simulink model "hh_ap"  (R2020b)
settings: Solver=VariableStepAuto  StartTime=0.0  StopTime=10.0  RelTol=1e-3
values from neighbouring files (symbols this model uses):
  capa = 1    [hh_ap_source.m]
  E_K = -12    [hh_ap_source.m]
  E_L = 10.613    [hh_ap_source.m]
  E_Na = 115    [hh_ap_source.m]
  G_K_max = 36    [hh_ap_source.m]
  G_L = 0.3    [hh_ap_source.m]
  G_Na_max = 120    [hh_ap_source.m]
  h0 = 1    [hh_ap_source.m]
  m0 = 0    [hh_ap_source.m]
  n0 = 0    [hh_ap_source.m]
  V0 = 0    [hh_ap_source.m]
settings Model: Creator=haedo  LastModifiedBy=haedo

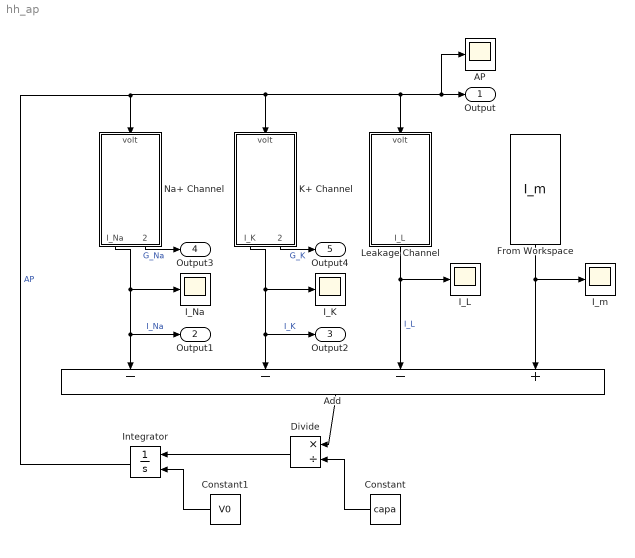
== system hh_ap ==
  AP : Scope
  Add : Sum  Inputs=---+
  Constant : Constant  Value=capa
  Constant1 : Constant  Value=V0
  Divide : Product  Inputs=*/
  From Workspace : FromWorkspace  VariableName=I_m
  I_K : Scope
  I_L : Scope
  I_Na : Scope
  I_m : Scope
  Integrator : Integrator  InitialConditionSource=external
  K+ Channel : Subsystem
  Leakage Channel : Subsystem
  Na+ Channel : Subsystem
  Output : Outport  VectorParamsAs1DForOutWhenUnconnected=off
  Output1 : Outport  Port=2  VectorParamsAs1DForOutWhenUnconnected=off
  Output2 : Outport  Port=3  VectorParamsAs1DForOutWhenUnconnected=off
  Output3 : Outport  Port=4  VectorParamsAs1DForOutWhenUnconnected=off
  Output4 : Outport  Port=5  VectorParamsAs1DForOutWhenUnconnected=off
  wires:
  Leakage Channel/1(I_L) -> I_L/1, Add/3  "I_L"
  Na+ Channel/2(G_Na_out) -> Output3/1  "G_Na"
  K+ Channel/2(G_K_out) -> Output4/1  "G_K"
  Constant1/1 -> Integrator/2
  Divide/1 -> Integrator/1
  Add/1 -> Divide/1
  Constant/1 -> Divide/2
  Na+ Channel/1(I_Na) -> I_Na/1, Output1/1, Add/1  "I_Na"
  Integrator/1 -> Na+ Channel/1(volt), AP/1, Output/1, Leakage Channel/1(volt), K+ Channel/1(volt)  "AP"
  K+ Channel/1(I_K) -> I_K/1, Output2/1, Add/2  "I_K"
  From Workspace/1 -> Add/4, I_m/1

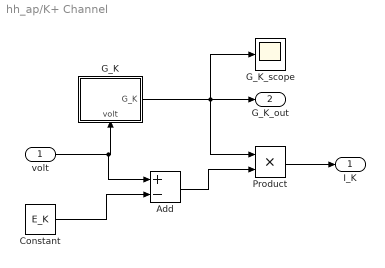
== system hh_ap/K+ Channel ==
  volt : Inport
  Add : Sum  Inputs=+-
  Constant : Constant  Value=E_K
  G_K : Subsystem
      settings: PortSchema="{\"entries\":[{\"content\":{\"sides\":[{\"content\":{\"connectorIds\":[]},\"type\":\"ConnectorPlacement.EquallySpacedRectSide\",\"uuid\":\"c632c91d-1676-4ce6-ab06-0028f8692ea5\"},{\"content\":{\"connectorIds\":[\"Out1\"],\"side\":\"RIGHT\"},\"type\":\"ConnectorPlacement.EquallySpacedRectSide\",\"uuid\":\"77b5085d-448e-4fc4-839b-3922e0b13526\"},{\"content\":{\"connectorIds\":[],\"side\":\"TOP\"},\"type\":\"ConnectorPlacement.EquallySpacedRectSide\",\"uuid\":\"dde0a616-523c-44d7-906e-d12cd1b401cf\"},{\"content\":{\"connectorIds\":[\"In1\"],\"side\":\"BOTTOM\"},\"type\":\"ConnectorPlacement.EquallySpacedRectSide\",\"uuid\":\"6c2ebf81-88aa-4156-83e6-a680f4cc31d9\"},{\"content\":{\"connectorIds\":[],\"side\":\"HIDDEN\"},\"type\":\"ConnectorPlacement.EquallySpacedRectSide\",\"uuid\":\"db869b89-d2b9-4524-8487-965b7fee0f2a\"}]},\"type\":\"ConnectorPlacement.EquallySpacedConnector\",\"uuid\":\"378f1207-81e2-4c7e-8dbf-20f9b4c806d5\"}],\"packageUris\":[\"http://schema.mathworks.com/mf0/Connector/R2020b\"],\"version\":\"1.0\"}"
  G_K_scope : Scope
  Product : Product
  I_K : Outport  VectorParamsAs1DForOutWhenUnconnected=off
  G_K_out : Outport  Port=2  VectorParamsAs1DForOutWhenUnconnected=off
  wires:
  volt/1 -> Add/1, G_K/1(volt)
  Constant/1 -> Add/2
  G_K/1(G_K) -> G_K_scope/1, G_K_out/1, Product/1
  Add/1 -> Product/2
  Product/1 -> I_K/1

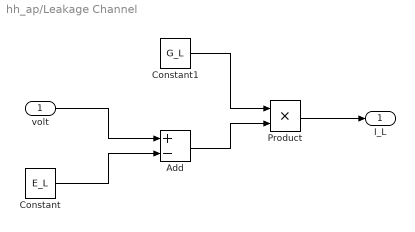
== system hh_ap/Leakage Channel ==
  volt : Inport
  Add : Sum  Inputs=+-
  Constant : Constant  Value=E_L
  Constant1 : Constant  Value=G_L
  Product : Product
  I_L : Outport  VectorParamsAs1DForOutWhenUnconnected=off
  wires:
  volt/1 -> Add/1
  Constant/1 -> Add/2
  Add/1 -> Product/2
  Constant1/1 -> Product/1
  Product/1 -> I_L/1

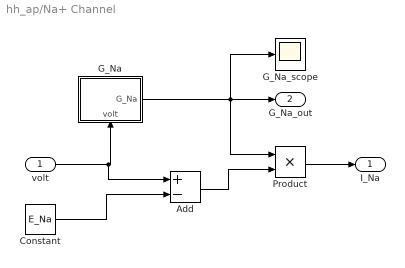
== system hh_ap/Na+ Channel ==
  volt : Inport
  Add : Sum  Inputs=+-
  Constant : Constant  Value=E_Na
  G_Na : Subsystem
      settings: PortSchema="{\"entries\":[{\"content\":{\"sides\":[{\"content\":{\"connectorIds\":[]},\"type\":\"ConnectorPlacement.EquallySpacedRectSide\",\"uuid\":\"c632c91d-1676-4ce6-ab06-0028f8692ea5\"},{\"content\":{\"connectorIds\":[\"Out1\"],\"side\":\"RIGHT\"},\"type\":\"ConnectorPlacement.EquallySpacedRectSide\",\"uuid\":\"77b5085d-448e-4fc4-839b-3922e0b13526\"},{\"content\":{\"connectorIds\":[],\"side\":\"TOP\"},\"type\":\"ConnectorPlacement.EquallySpacedRectSide\",\"uuid\":\"dde0a616-523c-44d7-906e-d12cd1b401cf\"},{\"content\":{\"connectorIds\":[\"In1\"],\"side\":\"BOTTOM\"},\"type\":\"ConnectorPlacement.EquallySpacedRectSide\",\"uuid\":\"c48f64ba-ba8f-42a4-9bef-aedab16ae96a\"},{\"content\":{\"connectorIds\":[],\"side\":\"HIDDEN\"},\"type\":\"ConnectorPlacement.EquallySpacedRectSide\",\"uuid\":\"db869b89-d2b9-4524-8487-965b7fee0f2a\"}]},\"type\":\"ConnectorPlacement.EquallySpacedConnector\",\"uuid\":\"378f1207-81e2-4c7e-8dbf-20f9b4c806d5\"}],\"packageUris\":[\"http://schema.mathworks.com/mf0/Connector/R2020b\"],\"version\":\"1.0\"}"
  G_Na_scope : Scope
  Product : Product
  I_Na : Outport  VectorParamsAs1DForOutWhenUnconnected=off
  G_Na_out : Outport  Port=2  VectorParamsAs1DForOutWhenUnconnected=off
  wires:
  volt/1 -> Add/1, G_Na/1(volt)
  Constant/1 -> Add/2
  G_Na/1(G_Na) -> G_Na_scope/1, G_Na_out/1, Product/1
  Add/1 -> Product/2
  Product/1 -> I_Na/1

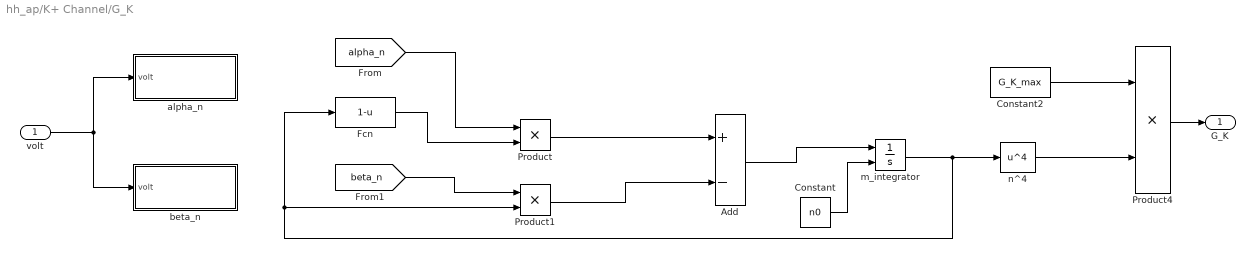
== system hh_ap/K+ Channel/G_K ==
  volt : Inport
  Add : Sum  Inputs=+-
  Constant : Constant  Value=n0
  Constant2 : Constant  Value=G_K_max
  Fcn : Fcn  Expr=1-u
  Product : Product
  Product1 : Product
  Product4 : Product
  alpha_n : Subsystem
  beta_n : Subsystem
  m_integrator : Integrator  InitialConditionSource=external
  n^4 : Fcn  Expr=u^4
  G_K : Outport
  wires:
  volt/1 -> alpha_n/1(volt), beta_n/1(volt)
  Product/1 -> Add/1
  [beta_n] -> Product1/1
  Add/1 -> m_integrator/1
  Product1/1 -> Add/2
  [alpha_n] -> Product/1
  Constant2/1 -> Product4/1
  n^4/1 -> Product4/2
  Product4/1 -> G_K/1
  m_integrator/1 -> n^4/1, Fcn/1, Product1/2
  Constant/1 -> m_integrator/2
  Fcn/1 -> Product/2

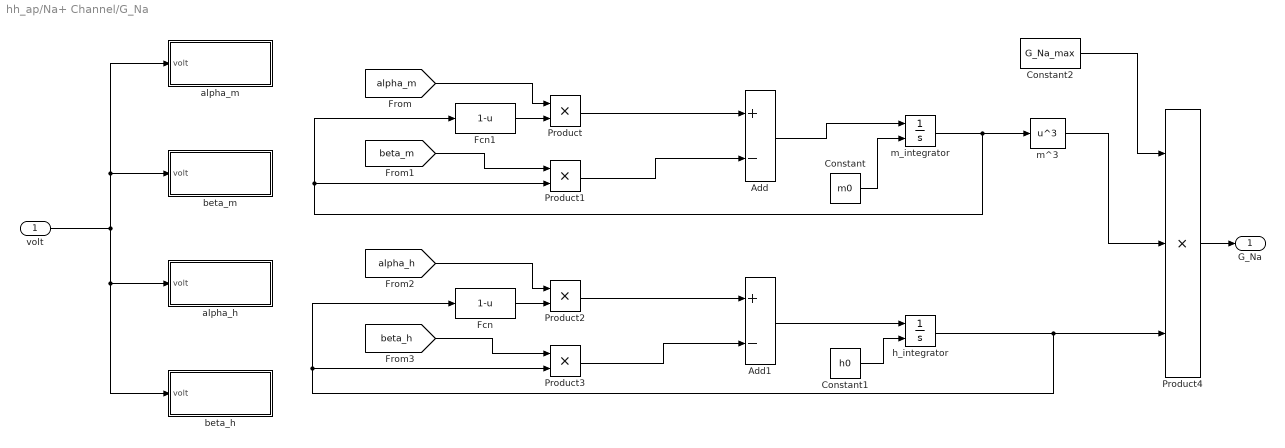
== system hh_ap/Na+ Channel/G_Na ==
  volt : Inport
  Add : Sum  Inputs=+-
  Add1 : Sum  Inputs=+-
  Constant : Constant  Value=m0
  Constant1 : Constant  Value=h0
  Constant2 : Constant  Value=G_Na_max
  Fcn : Fcn  Expr=1-u
  Fcn1 : Fcn  Expr=1-u
  Product{,1..3} (4 alike) : Product
  Product4 : Product  Inputs=3
  alpha_h : Subsystem
  alpha_m : Subsystem
  beta_h : Subsystem
  beta_m : Subsystem
  h_integrator : Integrator  InitialConditionSource=external
  m^3 : Fcn  Expr=u^3
  m_integrator : Integrator  InitialConditionSource=external
  G_Na : Outport
  wires:
  volt/1 -> beta_m/1(volt), alpha_m/1(volt), beta_h/1(volt), alpha_h/1(volt)
  h_integrator/1 -> Product3/2, Fcn/1, Product4/3
  m_integrator/1 -> m^3/1, Fcn1/1, Product1/2
  Fcn/1 -> Product2/2
  Fcn1/1 -> Product/2
  Product4/1 -> G_Na/1
  m^3/1 -> Product4/2
  Constant/1 -> m_integrator/2
  [beta_h] -> Product3/1
  Constant2/1 -> Product4/1
  Constant1/1 -> h_integrator/2
  [beta_m] -> Product1/1
  [alpha_h] -> Product2/1
  Product/1 -> Add/1
  Add1/1 -> h_integrator/1
  Product1/1 -> Add/2
  Product3/1 -> Add1/2
  Product2/1 -> Add1/1
  Add/1 -> m_integrator/1
  [alpha_m] -> Product/1

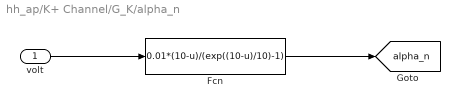
== system hh_ap/K+ Channel/G_K/alpha_n ==
  volt : Inport
  Fcn : Fcn  Expr=0.01*(10-u)/(exp((10-u)/10)-1)
  tag scope: alpha_n=global
  wires:
  Fcn/1 -> [alpha_n]
  volt/1 -> Fcn/1

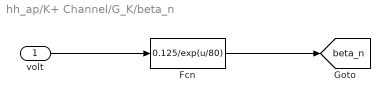
== system hh_ap/K+ Channel/G_K/beta_n ==
  volt : Inport
  Fcn : Fcn  Expr=0.125/exp(u/80)
  tag scope: beta_n=global
  wires:
  volt/1 -> Fcn/1
  Fcn/1 -> [beta_n]

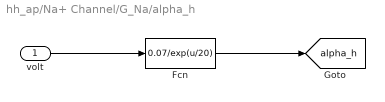
== system hh_ap/Na+ Channel/G_Na/alpha_h ==
  volt : Inport
  Fcn : Fcn  Expr=0.07/exp(u/20)
  tag scope: alpha_h=global
  wires:
  volt/1 -> Fcn/1
  Fcn/1 -> [alpha_h]

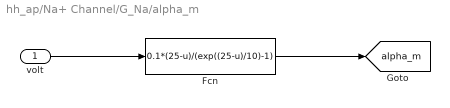
== system hh_ap/Na+ Channel/G_Na/alpha_m ==
  volt : Inport
  Fcn : Fcn  Expr=0.1*(25-u)/(exp((25-u)/10)-1)
  tag scope: alpha_m=global
  wires:
  Fcn/1 -> [alpha_m]
  volt/1 -> Fcn/1

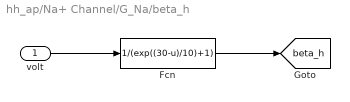
== system hh_ap/Na+ Channel/G_Na/beta_h ==
  volt : Inport
  Fcn : Fcn  Expr=1/(exp((30-u)/10)+1)
  tag scope: beta_h=global
  wires:
  volt/1 -> Fcn/1
  Fcn/1 -> [beta_h]

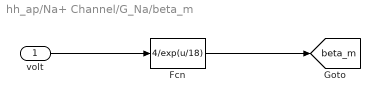
== system hh_ap/Na+ Channel/G_Na/beta_m ==
  volt : Inport
  Fcn : Fcn  Expr=4/exp(u/18)
  tag scope: beta_m=global
  wires:
  volt/1 -> Fcn/1
  Fcn/1 -> [beta_m]
